simulink model "sampleModel36"  (Simulink 9.1)
settings: Solver=VariableStepAuto  StartTime=0.0  StopTime=10.0  RelTol=1e-3
undefined symbols (not defined in the file): DiscIntNeverNeededParam, Newton, Raphson
libraries: simulink x48
(part 2 of 2)

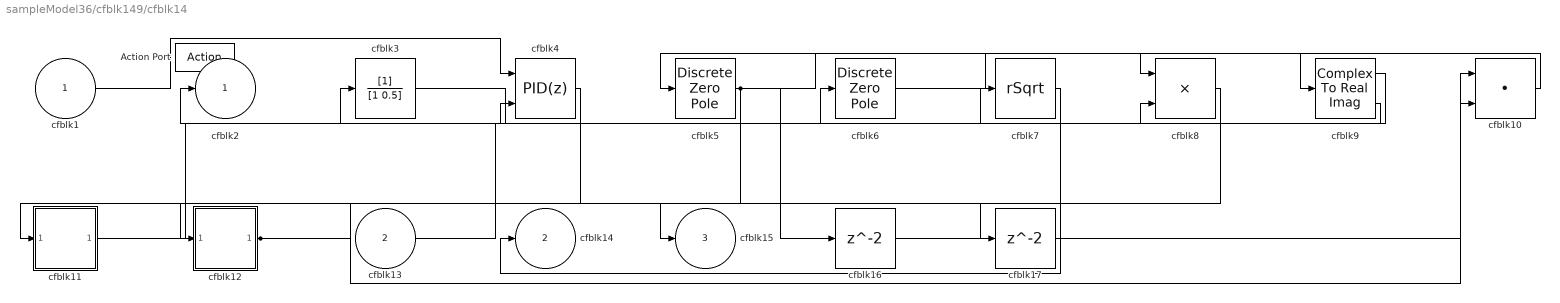
== system sampleModel36/cfblk149/cfblk14 ==
  cfblk1 : Inport
  cfblk13 : Inport  Port=2
  Action Port : ActionPort  ActionType=else
  cfblk10 : DotProduct  InputSameDT=on  OutDataTypeStr=Inherit: Inherit via internal rule
  cfblk11 : Subsystem
  cfblk12 : Subsystem
  cfblk16 : Delay
  cfblk17 : Delay
  cfblk3 : DiscreteFilter
  cfblk4 : simulink/Continuous/PID Controller (2DOF)  Controller=PID  TimeDomain=Discrete-time  SampleTime=-1  IntegratorMethod=Forward Euler  FilterMethod=Forward Euler  Form=Parallel  UseFilter=on  ControllerParametersSource=internal  P=1  I=1  D=0  N=100  b=1  c=1  InitialConditionSource=internal  InitialConditionForIntegrator=0  InitialConditionForFilter=0  ExternalReset=none  LimitOutput=off  UpperSaturationLimit=inf  LowerSaturationLimit=-inf  LinearizeAsGain=off  AntiWindupMode=none  Kb=1  TrackingMode=off  Kt=1  PParamMin=[]  PParamMax=[]  IParamMin=[]  IParamMax=[]  DParamMin=[]  DParamMax=[]  NParamMin=[]  NParamMax=[]  bParamMin=[]  bParamMax=[]  cParamMin=[]  cParamMax=[]  KbParamMin=[]  KbParamMax=[]  KtParamMin=[]  KtParamMax=[]  POutMin=[]  POutMax=[]  IOutMin=[]  IOutMax=[]  DOutMin=[]  DOutMax=[]  NOutMin=[]  NOutMax=[]  bOutMin=[]  bOutMax=[]  cOutMin=[]  cOutMax=[]  KbOutMin=[]  KbOutMax=[]  KtOutMin=[]  KtOutMax=[]  IntegratorOutMin=[]  IntegratorOutMax=[]  FilterOutMin=[]  FilterOutMax=[]  SumOutMin=[]  SumOutMax=[]  Sum1OutMin=[]  Sum1OutMax=[]  Sum2OutMin=[]  Sum2OutMax=[]  Sum3OutMin=[]  Sum3OutMax=[]  SumI1OutMin=[]  SumI1OutMax=[]  SumI2OutMin=[]  SumI2OutMax=[]  SumI3OutMin=[]  SumI3OutMax=[]  SumDOutMin=[]  SumDOutMax=[]  SaturationOutMin=[]  SaturationOutMax=[]  IntegratorContinuousStateAttributes=''  IntegratorStateMustResolveToSignalObject=off  IntegratorRTWStateStorageClass=Auto  FilterContinuousStateAttributes=''  FilterStateMustResolveToSignalObject=off  FilterRTWStateStorageClass=Auto  DifferentiatorICPrevScaledInput=0  DifferentiatorOutMin=[]  DifferentiatorOutMax=[]  FilterDiffOutCoefMin=[]  FilterDiffOutCoefMax=[]  SumDenOutMin=[]  SumDenOutMax=[]  SumNumOutMin=[]  SumNumOutMax=[]  ReciprocalOutMin=[]  ReciprocalOutMax=[]  DivideOutMin=[]  DivideOutMax=[]  TunerSelectOption=Transfer Function Based (PID Tuner App)
  cfblk5 : DiscreteZeroPole  Poles=[0 0.5]  Gain=1  SampleTime=-1
  cfblk6 : DiscreteZeroPole  Poles=[0 0.5]  Gain=1  SampleTime=-1
  cfblk7 : Sqrt  Operator=rSqrt  AlgorithmType=Newton-Raphson  SaturateOnIntegerOverflow=on
  cfblk8 : Product  Inputs=**
  cfblk9 : ComplexToRealImag
  cfblk2 : Outport
  cfblk14 : Outport  Port=2
  cfblk15 : Outport  Port=3
  wires:
  cfblk4/1 -> cfblk11/1(cfblk1)
  cfblk10/1 -> cfblk5/1
  cfblk7/1 -> cfblk14/1
  cfblk11/1(cfblk2) -> cfblk3/1
  cfblk6/1 -> cfblk8/1
  cfblk9/1 -> cfblk2/1
  cfblk12/1(cfblk2) -> cfblk10/1, cfblk17/1
  cfblk8/1 -> cfblk12/1(cfblk1)
  cfblk9/2 -> cfblk7/1
  cfblk1/1 -> cfblk4/1
  cfblk5/1 -> cfblk15/1, cfblk9/1, cfblk16/1
  cfblk3/1 -> cfblk6/1
  cfblk13/1 -> cfblk8/2
  cfblk16/1 -> cfblk10/2
  cfblk17/1 -> cfblk4/2

== system sampleModel36/cfblk149/cfblk15 ==
  cfblk1 : Inport
  Action Port : ActionPort  ActionType=then
  cfblk10 : Subsystem
  cfblk11 : Subsystem
  cfblk12 : Delay
  cfblk13 : Delay
  cfblk3 : Bias  Bias=[-449440720.085823]
  cfblk4 : Sqrt  Operator=rSqrt  AlgorithmType=Newton-Raphson  SaturateOnIntegerOverflow=on
  cfblk5 : PermuteDimensions
  cfblk6 : Reshape
  cfblk7 : Subsystem
  cfblk8 : Subsystem
  cfblk9 : Subsystem
  cfblk2 : Outport
  wires:
  cfblk7/1(cfblk2) -> cfblk11/1(cfblk1)
  cfblk6/1 -> cfblk10/1(cfblk1)
  cfblk3/1 -> cfblk4/1
  cfblk8/1(cfblk2) -> cfblk6/1
  cfblk11/1(cfblk2) -> cfblk2/1
  cfblk9/1(cfblk2) -> cfblk7/1(cfblk1)
  cfblk1/1 -> cfblk9/1(cfblk1)
  cfblk5/1 -> cfblk8/1(cfblk1)
  cfblk4/1 -> cfblk12/1
  cfblk12/1 -> cfblk3/1
  cfblk10/1(cfblk2) -> cfblk13/1
  cfblk13/1 -> cfblk5/1

== system sampleModel36/cfblk149/cfblk16 ==
  cfblk1 : Inport
  cfblk10 : Inport  Port=2
  cfblk11 : Inport  Port=3
  Action Port : ActionPort  ActionType=else
  cfblk3 : simulink/Discrete/Transfer Fcn Lead or Lag  PoleZ=0.95  ZeroZ=0.75  ICPrevOutput=0.0  ICPrevInput=0.0  DoSatur=off
      settings: SourceProductName=Simulink  SourceProductBaseCode=SL
  cfblk4 : Sum  Inputs=|++
  cfblk5 : Sin  TimeSource=Use external signal  SampleTime=0
  cfblk6 : Constant  Value=[-498528936.952922]  SampleTime=1
  cfblk7 : Subsystem
  cfblk8 : Subsystem
  cfblk9 : Subsystem
  cfblk2 : Outport
  cfblk12 : Outport  Port=2
  wires:
  cfblk9/1(cfblk2) -> cfblk5/1
  cfblk4/1 -> cfblk3/1
  cfblk11/1 -> cfblk8/1(cfblk1)
  cfblk5/1 -> cfblk4/1
  cfblk1/1 -> cfblk7/1(cfblk1)
  cfblk6/1 -> cfblk9/1(cfblk1)
  cfblk8/1(cfblk2) -> cfblk12/1
  cfblk10/1 -> cfblk4/2
  cfblk3/1 -> cfblk2/1

== system sampleModel36/cfblk149/cfblk7 ==
  cfblk1 : Inport
  cfblk2 : Outport
  wires:
  cfblk1/1 -> cfblk2/1

== system sampleModel36/cfblk149/cfblk8 ==
  cfblk1 : Inport
  cfblk2 : Outport
  wires:
  cfblk1/1 -> cfblk2/1

== system sampleModel36/cfblk150/cfblk10 ==
  cfblk1 : Inport
  cfblk2 : Outport
  wires:
  cfblk1/1 -> cfblk2/1

== system sampleModel36/cfblk150/cfblk11 ==
  cfblk1 : Inport
  cfblk2 : Outport
  wires:
  cfblk1/1 -> cfblk2/1

== system sampleModel36/cfblk150/cfblk12 ==
  cfblk1 : Inport
  cfblk2 : Outport
  wires:
  cfblk1/1 -> cfblk2/1

== system sampleModel36/cfblk150/cfblk7 ==
  cfblk1 : Inport
  cfblk2 : Outport
  wires:
  cfblk1/1 -> cfblk2/1

== system sampleModel36/cfblk150/cfblk8 ==
  cfblk1 : Inport
  cfblk2 : Outport
  wires:
  cfblk1/1 -> cfblk2/1

== system sampleModel36/cfblk150/cfblk9 ==
  cfblk1 : Inport
  cfblk2 : Outport
  wires:
  cfblk1/1 -> cfblk2/1

== system sampleModel36/cfblk152/cfblk6 ==
  cfblk1 : Inport
  cfblk2 : Outport
  wires:
  cfblk1/1 -> cfblk2/1

== system sampleModel36/cfblk152/cfblk7 ==
  cfblk1 : Inport
  cfblk2 : Outport
  wires:
  cfblk1/1 -> cfblk2/1

== system sampleModel36/cfblk153/cfblk11 ==
  cfblk1 : Inport
  cfblk2 : Outport
  wires:
  cfblk1/1 -> cfblk2/1

== system sampleModel36/cfblk153/cfblk12 ==
  cfblk1 : Inport
  cfblk2 : Outport
  wires:
  cfblk1/1 -> cfblk2/1

== system sampleModel36/cfblk154/cfblk9 ==
  cfblk1 : Inport
  cfblk2 : Outport
  wires:
  cfblk1/1 -> cfblk2/1

== system sampleModel36/cfblk155/cfblk11 ==
  cfblk1 : Inport
  cfblk2 : Outport
  wires:
  cfblk1/1 -> cfblk2/1

== system sampleModel36/cfblk155/cfblk12 ==
  cfblk1 : Inport
  cfblk2 : Outport
  wires:
  cfblk1/1 -> cfblk2/1

== system sampleModel36/cfblk156/cfblk10 ==
  cfblk1 : Inport
  cfblk2 : Outport
  wires:
  cfblk1/1 -> cfblk2/1

== system sampleModel36/cfblk156/cfblk8 ==
  cfblk1 : Inport
  cfblk2 : Outport
  wires:
  cfblk1/1 -> cfblk2/1

== system sampleModel36/cfblk156/cfblk9 ==
  cfblk1 : Inport
  cfblk2 : Outport
  wires:
  cfblk1/1 -> cfblk2/1

== system sampleModel36/cfblk157/cfblk10 ==
  cfblk1 : Inport
  cfblk2 : Outport
  wires:
  cfblk1/1 -> cfblk2/1

== system sampleModel36/cfblk157/cfblk11 ==
  cfblk1 : Inport
  cfblk2 : Outport
  wires:
  cfblk1/1 -> cfblk2/1

== system sampleModel36/cfblk157/cfblk9 ==
  cfblk1 : Inport
  cfblk2 : Outport
  wires:
  cfblk1/1 -> cfblk2/1

== system sampleModel36/cfblk158/cfblk10 ==
  cfblk1 : Inport
  cfblk2 : Outport
  wires:
  cfblk1/1 -> cfblk2/1

== system sampleModel36/cfblk158/cfblk11 ==
  cfblk1 : Inport
  cfblk2 : Outport
  wires:
  cfblk1/1 -> cfblk2/1

== system sampleModel36/cfblk158/cfblk12 ==
  cfblk1 : Inport
  cfblk2 : Outport
  wires:
  cfblk1/1 -> cfblk2/1

== system sampleModel36/cfblk158/cfblk13 ==
  cfblk1 : Inport
  cfblk2 : Outport
  wires:
  cfblk1/1 -> cfblk2/1

== system sampleModel36/cfblk158/cfblk8 ==
  cfblk1 : Inport
  cfblk2 : Outport
  wires:
  cfblk1/1 -> cfblk2/1

== system sampleModel36/cfblk158/cfblk9 ==
  cfblk1 : Inport
  cfblk2 : Outport
  wires:
  cfblk1/1 -> cfblk2/1

== system sampleModel36/cfblk159/cfblk13 ==
  cfblk1 : Inport
  cfblk2 : Outport
  wires:
  cfblk1/1 -> cfblk2/1

== system sampleModel36/cfblk159/cfblk14 ==
  cfblk1 : Inport
  cfblk2 : Outport
  wires:
  cfblk1/1 -> cfblk2/1

== system sampleModel36/cfblk159/cfblk15 ==
  cfblk1 : Inport
  cfblk2 : Outport
  wires:
  cfblk1/1 -> cfblk2/1

== system sampleModel36/cfblk159/cfblk16 ==
  cfblk1 : Inport
  cfblk2 : Outport
  wires:
  cfblk1/1 -> cfblk2/1

== system sampleModel36/cfblk160/cfblk12 ==
  cfblk1 : Inport
  cfblk2 : Outport
  wires:
  cfblk1/1 -> cfblk2/1

== system sampleModel36/cfblk161/cfblk11 ==
  cfblk1 : Inport
  cfblk8 : Inport  Port=2
  cfblk9 : Inport  Port=3
  Action Port : ActionPort  ActionType=then
  cfblk10 : Delay
  cfblk3 : Delay  DelayLengthSource=Input port
      settings: InputPortMap=u0,p1
  cfblk4 : DiscreteZeroPole  Poles=[0 0.5]  Gain=1  SampleTime=-1
  cfblk5 : simulink/Math Operations/Slider Gain  gain=1  low=0  high=2
  cfblk6 : Product  Inputs=*
  cfblk7 : Constant  Value=[208722222.162422]  SampleTime=1
  cfblk2 : Outport
  wires:
  cfblk9/1 -> cfblk5/1
  cfblk3/1 -> cfblk6/1
  cfblk1/1 -> cfblk2/1
  cfblk4/1 -> cfblk3/1
  cfblk7/1 -> cfblk4/1
  cfblk6/1 -> cfblk10/1
  cfblk10/1 -> cfblk3/2

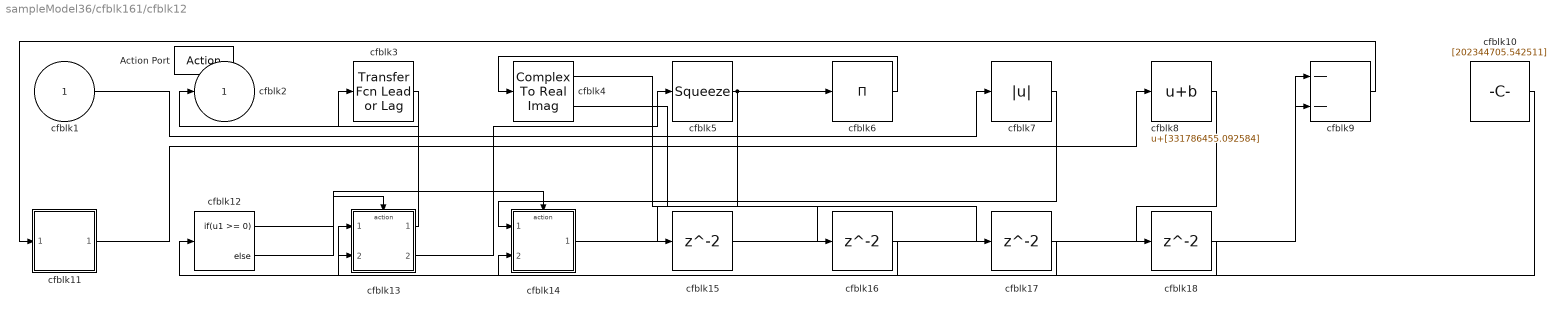
== system sampleModel36/cfblk161/cfblk12 ==
  cfblk1 : Inport
  Action Port : ActionPort  ActionType=else
  cfblk10 : Constant  Value=[202344705.542511]  SampleTime=1
  cfblk11 : Subsystem
  cfblk12 : If  IfExpression=u1 >= 0  SampleTime=1
  cfblk13 : Subsystem  TreatAsAtomicUnit=on
  cfblk14 : Subsystem  TreatAsAtomicUnit=on
  cfblk{15..18} (4 alike) : Delay
  cfblk3 : simulink/Discrete/Transfer Fcn Lead or Lag  PoleZ=0.95  ZeroZ=0.75  ICPrevOutput=0.0  ICPrevInput=0.0  DoSatur=off
      settings: SourceProductName=Simulink  SourceProductBaseCode=SL
  cfblk4 : ComplexToRealImag
  cfblk5 : Squeeze
  cfblk6 : Product  Inputs=*
  cfblk7 : Abs
  cfblk8 : Bias  Bias=[331786455.092584]
  cfblk9 : Sum  Inputs=--
  cfblk2 : Outport
  wires:
  cfblk6/1 -> cfblk4/1
  cfblk3/1 -> cfblk2/1
  cfblk1/1 -> cfblk7/1
  cfblk11/1(cfblk2) -> cfblk8/1
  cfblk10/1 -> cfblk13/1(cfblk1)
  cfblk7/1 -> cfblk14/1(cfblk1)
  cfblk14/1(cfblk2) -> cfblk9/1
  cfblk9/1 -> cfblk11/1(cfblk1)
  cfblk5/1 -> cfblk6/1, cfblk15/1
  cfblk13/1(cfblk2) -> cfblk3/1
  cfblk13/2(cfblk8) -> cfblk5/1
  cfblk12/1 -> cfblk13/Action
  cfblk12/2 -> cfblk14/Action
  cfblk15/1 -> cfblk9/2
  cfblk4/1 -> cfblk16/1
  cfblk16/1 -> cfblk13/2(cfblk7)
  cfblk4/2 -> cfblk17/1
  cfblk17/1 -> cfblk14/2(cfblk7)
  cfblk8/1 -> cfblk18/1
  cfblk18/1 -> cfblk12/1

== system sampleModel36/cfblk161/cfblk6 ==
  cfblk1 : Inport
  cfblk2 : Outport
  wires:
  cfblk1/1 -> cfblk2/1

== system sampleModel36/cfblk161/cfblk7 ==
  cfblk1 : Inport
  cfblk2 : Outport
  wires:
  cfblk1/1 -> cfblk2/1

== system sampleModel36/cfblk162/cfblk5 ==
  cfblk1 : Inport
  cfblk2 : Outport
  wires:
  cfblk1/1 -> cfblk2/1

== system sampleModel36/cfblk162/cfblk6 ==
  cfblk1 : Inport
  cfblk2 : Outport
  wires:
  cfblk1/1 -> cfblk2/1

== system sampleModel36/cfblk162/cfblk7 ==
  cfblk1 : Inport
  cfblk2 : Outport
  wires:
  cfblk1/1 -> cfblk2/1

== system sampleModel36/cfblk163/cfblk13 ==
  cfblk1 : Inport
  cfblk2 : Outport
  wires:
  cfblk1/1 -> cfblk2/1

== system sampleModel36/cfblk163/cfblk14 ==
  cfblk1 : Inport
  cfblk2 : Outport
  wires:
  cfblk1/1 -> cfblk2/1

== system sampleModel36/cfblk163/cfblk15 ==
  cfblk1 : Inport
  cfblk2 : Outport
  wires:
  cfblk1/1 -> cfblk2/1

== system sampleModel36/cfblk164/cfblk5 ==
  cfblk1 : Inport
  cfblk2 : Outport
  wires:
  cfblk1/1 -> cfblk2/1

== system sampleModel36/cfblk164/cfblk6 ==
  cfblk1 : Inport
  cfblk2 : Outport
  wires:
  cfblk1/1 -> cfblk2/1

== system sampleModel36/cfblk164/cfblk7 ==
  cfblk1 : Inport
  cfblk2 : Outport
  wires:
  cfblk1/1 -> cfblk2/1

== system sampleModel36/cfblk149/cfblk13/cfblk6 ==
  cfblk1 : Inport
  cfblk2 : Outport
  wires:
  cfblk1/1 -> cfblk2/1

== system sampleModel36/cfblk149/cfblk13/cfblk7 ==
  cfblk1 : Inport
  cfblk2 : Outport
  wires:
  cfblk1/1 -> cfblk2/1

== system sampleModel36/cfblk149/cfblk13/cfblk8 ==
  cfblk1 : Inport
  cfblk2 : Outport
  wires:
  cfblk1/1 -> cfblk2/1

== system sampleModel36/cfblk149/cfblk13/cfblk9 ==
  cfblk1 : Inport
  cfblk2 : Outport
  wires:
  cfblk1/1 -> cfblk2/1

== system sampleModel36/cfblk149/cfblk14/cfblk11 ==
  cfblk1 : Inport
  cfblk2 : Outport
  wires:
  cfblk1/1 -> cfblk2/1

== system sampleModel36/cfblk149/cfblk14/cfblk12 ==
  cfblk1 : Inport
  cfblk2 : Outport
  wires:
  cfblk1/1 -> cfblk2/1

== system sampleModel36/cfblk149/cfblk15/cfblk10 ==
  cfblk1 : Inport
  cfblk2 : Outport
  wires:
  cfblk1/1 -> cfblk2/1

== system sampleModel36/cfblk149/cfblk15/cfblk11 ==
  cfblk1 : Inport
  cfblk2 : Outport
  wires:
  cfblk1/1 -> cfblk2/1

== system sampleModel36/cfblk149/cfblk15/cfblk7 ==
  cfblk1 : Inport
  cfblk2 : Outport
  wires:
  cfblk1/1 -> cfblk2/1

== system sampleModel36/cfblk149/cfblk15/cfblk8 ==
  cfblk1 : Inport
  cfblk2 : Outport
  wires:
  cfblk1/1 -> cfblk2/1

== system sampleModel36/cfblk149/cfblk15/cfblk9 ==
  cfblk1 : Inport
  cfblk2 : Outport
  wires:
  cfblk1/1 -> cfblk2/1

== system sampleModel36/cfblk149/cfblk16/cfblk7 ==
  cfblk1 : Inport
  cfblk2 : Outport
  wires:
  cfblk1/1 -> cfblk2/1

== system sampleModel36/cfblk149/cfblk16/cfblk8 ==
  cfblk1 : Inport
  cfblk2 : Outport
  wires:
  cfblk1/1 -> cfblk2/1

== system sampleModel36/cfblk149/cfblk16/cfblk9 ==
  cfblk1 : Inport
  cfblk2 : Outport
  wires:
  cfblk1/1 -> cfblk2/1

== system sampleModel36/cfblk161/cfblk12/cfblk11 ==
  cfblk1 : Inport
  cfblk2 : Outport
  wires:
  cfblk1/1 -> cfblk2/1

== system sampleModel36/cfblk161/cfblk12/cfblk13 ==
  cfblk1 : Inport
  cfblk7 : Inport  Port=2
  Action Port : ActionPort  ActionType=then
  cfblk10 : Subsystem  TreatAsAtomicUnit=on
  cfblk11 : Delay
  cfblk12 : Delay
  cfblk3 : simulink/Discrete/Transfer Fcn Lead or Lag  PoleZ=0.95  ZeroZ=0.75  ICPrevOutput=0.0  ICPrevInput=0.0  DoSatur=off
      settings: SourceProductName=Simulink  SourceProductBaseCode=SL
  cfblk4 : Constant  Value=[-702884140.949600]  SampleTime=1
  cfblk5 : Subsystem
  cfblk6 : If  IfExpression=u1 >= 0  SampleTime=1
  cfblk9 : Subsystem  TreatAsAtomicUnit=on
  cfblk2 : Outport
  cfblk8 : Outport  Port=2
  wires:
  cfblk4/1 -> cfblk5/1(cfblk1), cfblk9/4(cfblk14)
  cfblk7/1 -> cfblk10/1(cfblk1)
  cfblk5/1(cfblk2) -> cfblk9/1(cfblk1), cfblk10/4(cfblk9)
  cfblk10/1(cfblk2) -> cfblk3/1
  cfblk10/2(cfblk10) -> cfblk2/1
  cfblk9/1(cfblk2) -> cfblk8/1
  cfblk1/1 -> cfblk9/2(cfblk12), cfblk6/1
  cfblk3/1 -> cfblk11/1, cfblk12/1
  cfblk9/2(cfblk15) -> cfblk10/2(cfblk7)
  cfblk6/1 -> cfblk9/Action
  cfblk6/2 -> cfblk10/Action
  cfblk11/1 -> cfblk9/3(cfblk13)
  cfblk12/1 -> cfblk10/3(cfblk8)

== system sampleModel36/cfblk161/cfblk12/cfblk14 ==
  cfblk1 : Inport
  cfblk7 : Inport  Port=2
  Action Port : ActionPort  ActionType=else
  cfblk3 : UnitDelay  SampleTime=-1
  cfblk4 : Subsystem
  cfblk5 : Subsystem
  cfblk6 : Subsystem
  cfblk2 : Outport
  wires:
  cfblk1/1 -> cfblk6/1(cfblk1)
  cfblk5/1(cfblk2) -> cfblk4/1(cfblk1)
  cfblk7/1 -> cfblk3/1
  cfblk6/1(cfblk2) -> cfblk5/1(cfblk1)
  cfblk3/1 -> cfblk2/1

== system sampleModel36/cfblk161/cfblk12/cfblk13/cfblk10 ==
  cfblk1 : Inport
  cfblk7 : Inport  Port=2
  cfblk8 : Inport  Port=3
  cfblk9 : Inport  Port=4
  Action Port : ActionPort  ActionType=else
  cfblk3 : DiscreteFir
  cfblk4 : Delay  DelayLengthSource=Input port
      settings: InputPortMap=u0,p1
  cfblk5 : UnitDelay  SampleTime=-1
  cfblk6 : Product
  cfblk2 : Outport
  cfblk10 : Outport  Port=2
  wires:
  cfblk3/1 -> cfblk10/1
  cfblk9/1 -> cfblk6/1
  cfblk6/1 -> cfblk2/1
  cfblk8/1 -> cfblk5/1
  cfblk1/1 -> cfblk6/2
  cfblk4/1 -> cfblk3/1
  cfblk7/1 -> cfblk4/1
  cfblk5/1 -> cfblk4/2

== system sampleModel36/cfblk161/cfblk12/cfblk13/cfblk5 ==
  cfblk1 : Inport
  cfblk2 : Outport
  wires:
  cfblk1/1 -> cfblk2/1

== system sampleModel36/cfblk161/cfblk12/cfblk13/cfblk9 ==
  cfblk1 : Inport
  cfblk12 : Inport  Port=2
  cfblk13 : Inport  Port=3
  cfblk14 : Inport  Port=4
  Action Port : ActionPort  ActionType=then
  cfblk10 : Constant  Value=[-614816836.896723]  SampleTime=1
  cfblk11 : Constant  Value=[-344585341.652651]  SampleTime=1
  cfblk3 : simulink/Continuous/PID Controller (2DOF)  Controller=PID  TimeDomain=Discrete-time  SampleTime=-1  IntegratorMethod=Forward Euler  FilterMethod=Forward Euler  Form=Parallel  UseFilter=on  ControllerParametersSource=internal  P=1  I=1  D=0  N=100  b=1  c=1  InitialConditionSource=internal  InitialConditionForIntegrator=0  InitialConditionForFilter=0  ExternalReset=none  LimitOutput=off  UpperSaturationLimit=inf  LowerSaturationLimit=-inf  LinearizeAsGain=off  AntiWindupMode=none  Kb=1  TrackingMode=off  Kt=1  PParamMin=[]  PParamMax=[]  IParamMin=[]  IParamMax=[]  DParamMin=[]  DParamMax=[]  NParamMin=[]  NParamMax=[]  bParamMin=[]  bParamMax=[]  cParamMin=[]  cParamMax=[]  KbParamMin=[]  KbParamMax=[]  KtParamMin=[]  KtParamMax=[]  POutMin=[]  POutMax=[]  IOutMin=[]  IOutMax=[]  DOutMin=[]  DOutMax=[]  NOutMin=[]  NOutMax=[]  bOutMin=[]  bOutMax=[]  cOutMin=[]  cOutMax=[]  KbOutMin=[]  KbOutMax=[]  KtOutMin=[]  KtOutMax=[]  IntegratorOutMin=[]  IntegratorOutMax=[]  FilterOutMin=[]  FilterOutMax=[]  SumOutMin=[]  SumOutMax=[]  Sum1OutMin=[]  Sum1OutMax=[]  Sum2OutMin=[]  Sum2OutMax=[]  Sum3OutMin=[]  Sum3OutMax=[]  SumI1OutMin=[]  SumI1OutMax=[]  SumI2OutMin=[]  SumI2OutMax=[]  SumI3OutMin=[]  SumI3OutMax=[]  SumDOutMin=[]  SumDOutMax=[]  SaturationOutMin=[]  SaturationOutMax=[]  IntegratorContinuousStateAttributes=''  IntegratorStateMustResolveToSignalObject=off  IntegratorRTWStateStorageClass=Auto  FilterContinuousStateAttributes=''  FilterStateMustResolveToSignalObject=off  FilterRTWStateStorageClass=Auto  DifferentiatorICPrevScaledInput=0  DifferentiatorOutMin=[]  DifferentiatorOutMax=[]  FilterDiffOutCoefMin=[]  FilterDiffOutCoefMax=[]  SumDenOutMin=[]  SumDenOutMax=[]  SumNumOutMin=[]  SumNumOutMax=[]  ReciprocalOutMin=[]  ReciprocalOutMax=[]  DivideOutMin=[]  DivideOutMax=[]  TunerSelectOption=Transfer Function Based (PID Tuner App)
  cfblk4 : Math  Operator=pow  SaturateOnIntegerOverflow=on
  cfblk5 : Sum  Inputs=+
  cfblk6 : ComplexToMagnitudeAngle
  cfblk7 : Sum  Inputs=+-
  cfblk8 : Product  Inputs=**
  cfblk9 : Constant  Value=[-740987452.287222]  SampleTime=1
  cfblk2 : Outport
  cfblk15 : Outport  Port=2
  wires:
  cfblk11/1 -> cfblk3/1
  cfblk9/1 -> cfblk3/2
  cfblk3/1 -> cfblk6/1
  cfblk14/1 -> cfblk7/1
  cfblk6/1 -> cfblk7/2
  cfblk10/1 -> cfblk2/1
  cfblk7/1 -> cfblk5/1
  cfblk8/1 -> cfblk4/1
  cfblk5/1 -> cfblk4/2
  cfblk6/2 -> cfblk15/1
  cfblk1/1 -> cfblk8/1
  cfblk13/1 -> cfblk8/2

== system sampleModel36/cfblk161/cfblk12/cfblk14/cfblk4 ==
  cfblk1 : Inport
  cfblk2 : Outport
  wires:
  cfblk1/1 -> cfblk2/1

== system sampleModel36/cfblk161/cfblk12/cfblk14/cfblk5 ==
  cfblk1 : Inport
  cfblk2 : Outport
  wires:
  cfblk1/1 -> cfblk2/1

== system sampleModel36/cfblk161/cfblk12/cfblk14/cfblk6 ==
  cfblk1 : Inport
  cfblk2 : Outport
  wires:
  cfblk1/1 -> cfblk2/1
